simulink model "mars_para"  (R2022b)
settings: Solver=VariableStepDiscrete  StartTime=0.0  StopTime=200  RelTol=1e-3  EnableMultiTasking=on
PreLoadFcn:
  | % Input data
  | load mars_para_data
libraries: simulink x3
settings Model: Creator=nicholas  LastModifiedBy=bensweet
settings SolverCC: AlgebraicLoopSolver=TrustRegion  AutoInsertRateTranBlk=on
settings DataIOCC: ExternalInput=[t, Alt, Vel]  LoadExternalInput=on  SaveFormat=Array  ReturnWorkspaceOutputs=off
settings OptimizationCC: ExpressionDepthLimit=2147483647  InitFltsAndDblsToZero=on  LifeSpan=1  EfficientTunableParamExpr=on
settings DebuggingCC: UnconnectedInputMsg=warning  UnconnectedOutputMsg=warning  UnconnectedLineMsg=warning  PregeneratedLibrarySubsystemCodeDiagnostic=none  SFMachineParentedDataDiag=warning
settings HardwareCC: ProdBitPerPointer=32  ProdBitPerSizeT=32  ProdBitPerPtrDiffT=32  ProdLargestAtomicFloat=None  ProdIntDivRoundTo=Undefined  ProdEndianess=Unspecified  ProdWordSize=32  ProdHWDeviceType=32-bit Generic
settings ModelReferenceCC: EnableRefExpFcnMdlSchedulingChecks=on  PropagateSignalLabelsOutOfModel=off
settings SFSimCC: SimUseLocalCustomCode=off  SimParseCustomCode=off  MATLABDynamicMemAlloc=off
settings RTWCC: Description=RTW Embedded Coder (no auto configuration)  SystemTargetFile=ert.tlc  GenCodeOnly=on  TemplateMakefile=ert_default_tmf  RTWUseLocalCustomCode=off  DLArmComputeVersion=19.05
settings CodeAppCC: IgnoreCustomStorageClasses=off  CustomSymbolStrType=$N$R$M  StateflowObjectComments=on  InternalIdentifier=Classic
settings ERTTargetCC: TargetFcnLib=ansi_tfl_tmw.mat  MultiwordLength=2048  GenerateSampleERTMain=on  ERTCustomFileTemplate=example_file_process.tlc  ConvertIfToSwitch=off  SuppressUnreachableDefaultCases=off
settings ConfigComp: CovMetricSettings=dw  CovSaveCumulativeToWorkspaceVar=on  CovSaveSingleToWorkspaceVar=on  CovExternalEMLEnable=off  CovSFcnEnable=off

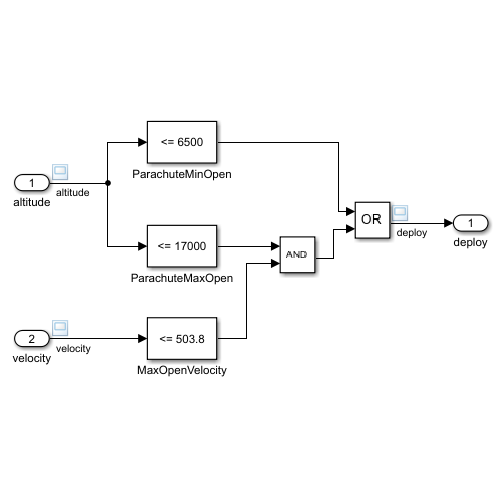
[thumbnail: Simulink's stored preview of the top-level diagram]
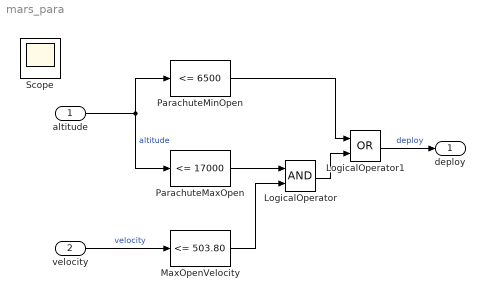
== system mars_para ==
  altitude : Inport
  velocity : Inport  Port=2
  LogicalOperator : Logic  AllPortsSameDT=off  OutDataTypeStr=boolean
  LogicalOperator1 : Logic  Operator=OR  AllPortsSameDT=off  OutDataTypeStr=boolean
  MaxOpenVelocity : simulink/Logic and Bit Operations/Compare To Constant  relop=<=  const=503.80  OutDataTypeStr=boolean
  ParachuteMaxOpen : simulink/Logic and Bit Operations/Compare To Constant  relop=<=  const=17000  OutDataTypeStr=boolean
  ParachuteMinOpen : simulink/Logic and Bit Operations/Compare To Constant  relop=<=  const=6500  OutDataTypeStr=boolean
  deploy : Outport  VectorParamsAs1DForOutWhenUnconnected=off
  Scope : Scope
  wires:
  LogicalOperator1/1 -> deploy/1  "deploy"
  altitude/1 -> ParachuteMinOpen/1, ParachuteMaxOpen/1  "altitude"
  ParachuteMaxOpen/1 -> LogicalOperator/1
  velocity/1 -> MaxOpenVelocity/1  "velocity"
  MaxOpenVelocity/1 -> LogicalOperator/2
  ParachuteMinOpen/1 -> LogicalOperator1/1
  LogicalOperator/1 -> LogicalOperator1/2
